simulink library "Angle_Wrap_lib"  (R2023a)
settings: Solver=VariableStepAuto  StartTime=0.0  StopTime=10.0  RelTol=1e-3
libraries: simulink_extras x3, Rotation2D x1
settings Model: Creator=ander  LastModifiedBy=ander

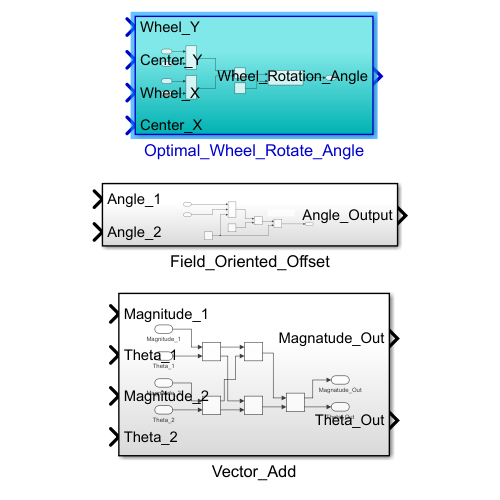
[thumbnail: Simulink's stored preview of the top-level diagram]
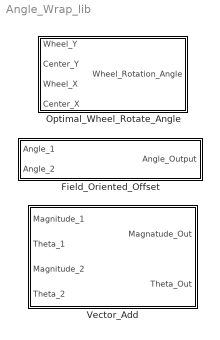
== system Angle_Wrap_lib ==
  Field_Oriented_Offset : Subsystem
  Optimal_Wheel_Rotate_Angle : Subsystem
  Vector_Add : Subsystem

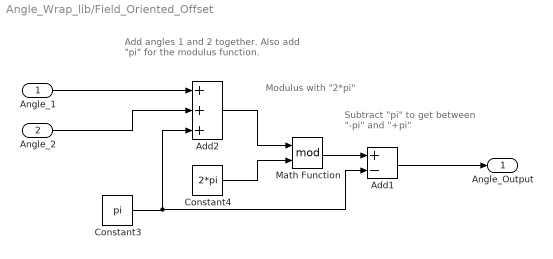
== system Angle_Wrap_lib/Field_Oriented_Offset ==
  note: Add angles 1 and 2 together.
      | Also add "pi" for the modulus function.
  note: Modulus with "2*pi"
  note: Subtract "pi" to get
      | between "-pi" and "+pi"
  Angle_1 : Inport
  Angle_2 : Inport  Port=2
  Add1 : Sum  Inputs=+-
  Add2 : Sum  Inputs=3
  Constant3 : Constant  Value=pi
  Constant4 : Constant  Value=2*pi
  Math Function : Math  Operator=mod
  Angle_Output : Outport
  wires:
  Angle_1/1 -> Add2/1
  Constant3/1 -> Add2/3, Add1/2
  Add2/1 -> Math Function/1
  Constant4/1 -> Math Function/2
  Math Function/1 -> Add1/1
  Add1/1 -> Angle_Output/1
  Angle_2/1 -> Add2/2

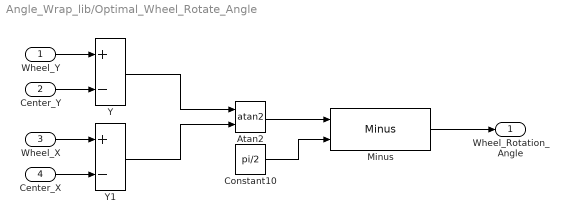
== system Angle_Wrap_lib/Optimal_Wheel_Rotate_Angle ==
  Wheel_Y : Inport
  Center_Y : Inport  Port=2
  Wheel_X : Inport  Port=3
  Center_X : Inport  Port=4
  Atan2 : Trigonometry  Operator=atan2
  Constant10 : Constant  Value=pi/2
  Minus : Rotation2D/Minus  SystemSampleTime=-1  VariantActivationTime=update diagram  Latency=0  AutoFrameSizeCalculation=off
  Y : Sum  Inputs=+-
  Y1 : Sum  Inputs=+-
  Wheel_Rotation_Angle : Outport
  wires:
  Atan2/1 -> Minus/1
  Constant10/1 -> Minus/2
  Y/1 -> Atan2/1
  Y1/1 -> Atan2/2
  Minus/1 -> Wheel_Rotation_Angle/1
  Wheel_Y/1 -> Y/1
  Center_Y/1 -> Y/2
  Wheel_X/1 -> Y1/1
  Center_X/1 -> Y1/2

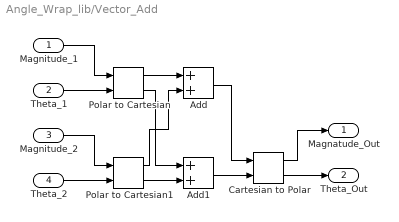
== system Angle_Wrap_lib/Vector_Add ==
  Magnitude_1 : Inport
  Theta_1 : Inport  Port=2
  Magnitude_2 : Inport  Port=3
  Theta_2 : Inport  Port=4
  Add : Sum
  Add1 : Sum
  Cartesian to Polar : simulink_extras/Transformations/Cartesian to Polar
  Polar to Cartesian : simulink_extras/Transformations/Polar to Cartesian
  Polar to Cartesian1 : simulink_extras/Transformations/Polar to Cartesian
  Magnatude_Out : Outport
  Theta_Out : Outport  Port=2
  wires:
  Magnitude_1/1 -> Polar to Cartesian/1
  Polar to Cartesian1/1 -> Add/2
  Polar to Cartesian/2 -> Add1/1
  Magnitude_2/1 -> Polar to Cartesian1/1
  Theta_1/1 -> Polar to Cartesian/2
  Polar to Cartesian/1 -> Add/1
  Polar to Cartesian1/2 -> Add1/2
  Theta_2/1 -> Polar to Cartesian1/2
  Add/1 -> Cartesian to Polar/1
  Add1/1 -> Cartesian to Polar/2
  Cartesian to Polar/1 -> Magnatude_Out/1
  Cartesian to Polar/2 -> Theta_Out/1
